simulink model "NestedEMF"  (Simulink 7.4)
settings: Solver=ode45  StartTime=0.0  StopTime=10.0  RelTol=1e-3
settings Model: Creator=dread  LastModifiedBy=dread

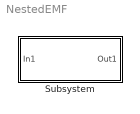
== system NestedEMF ==
  Subsystem : Subsystem

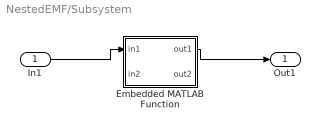
== system NestedEMF/Subsystem ==
  In1 : Inport  OutDataType=fixdt(1, 16)  OutScaling=2^0
  Embedded MATLAB Function : Stateflow chart
  Out1 : Outport  OutDataType=fixdt(1, 16)  OutScaling=2^0
  wires:
  In1/1 -> Embedded MATLAB Function/1(in1)
  Embedded MATLAB Function/1(out1) -> Out1/1

== matlab function Subsystem/Embedded MATLAB Function ==
  data: in1 input double; out1 output double; out2 output double; in2 input double
function [out1, out2] = fcn(in1, in2)
%#eml
out1 = in1;
out2 = in2;
